simulink model "savareseC2"  (R2023a)
settings: Solver=FixedStepDiscrete  StartTime=0.0  StopTime=200  FixedStep=Ts  MaxStep=Ts  RelTol=1e-3
model workspace (MAT data in the model file):
  Ts = 0.002
  acoeff = 0.95
  amax = 0.1
  jcoeff = 0.1
  jmax = 1
  pf = 160
  reference_command = [0 0.002 0.004 0.006 0.008 0.01 0.012 0.014 0.016 0.018 0.02 0.022 ... (200002 elements, 100001x2)]
  v = 50
  vmax = 1.5
undefined symbols (not defined in the file or in its folder): DiscIntNeverNeededParam
(part 1 of 2)
settings Model: Creator=savar  LastModifiedBy=giaco
settings SolverCC: AlgebraicLoopSolver=TrustRegion
settings DebuggingCC: UnconnectedInputMsg=warning  UnconnectedOutputMsg=warning  UnconnectedLineMsg=warning
settings ModelReferenceCC: EnableRefExpFcnMdlSchedulingChecks=on
settings RTWCC: DLArmComputeVersion=19.05

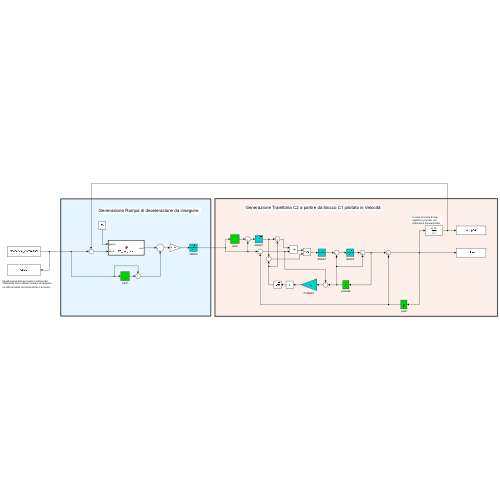
[thumbnail: Simulink's stored preview of the top-level diagram]
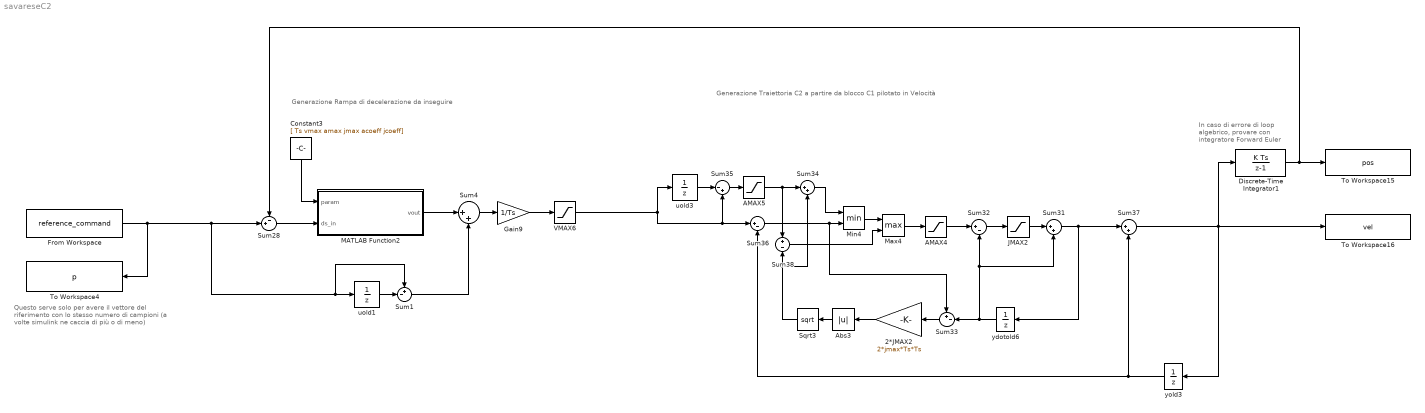
== system savareseC2 ==
  note: Questo serve solo per avere il vettore del riferimento con lo stesso numero di campioni
      | (a volte simulink ne caccia di più o di meno)
  note: In caso di errore di loop algebrico, provare con integratore Forward Euler
  note: Generazione Traiettoria C2 a partire da blocco C1 pilotato in Velocità
  note: Generazione Rampa di decelerazione da inseguire
  2*JMAX2 : Gain  Gain=2*jmax*Ts*Ts
  AMAX4 : Saturate  UpperLimit=amax*Ts  LowerLimit=-amax*Ts
  AMAX5 : Saturate  UpperLimit=amax*Ts  LowerLimit=-amax*Ts
  Abs3 : Abs  SaturateOnIntegerOverflow=off
  Constant3 : Constant  Value=[ Ts vmax amax jmax acoeff jcoeff]
  Discrete-Time Integrator1 : DiscreteIntegrator  SampleTime=-1  ICPrevOutput=DiscIntNeverNeededParam  ICPrevScaledInput=DiscIntNeverNeededParam
  From Workspace : FromWorkspace  VariableName=reference_command
  Gain9 : Gain  Gain=1/Ts
  JMAX2 : Saturate  UpperLimit=jmax*Ts*Ts  LowerLimit=-jmax*Ts*Ts
  MATLAB Function2 : MATLAB Function  TreatAsAtomicUnit=on
  Max4 : MinMax  Function=max  Inputs=2
  Min4 : MinMax  Inputs=2
  Sqrt3 : Sqrt
  Sum1 : Sum  Inputs=+-|
  Sum28 : Sum  Inputs=-+|
  Sum{4,31,34,37} (4 alike) : Sum  Inputs=|++
  Sum32 : Sum  Inputs=|+-
  Sum33 : Sum  Inputs=+-|
  Sum35 : Sum  Inputs=|-+
  Sum36 : Sum  Inputs=|+-
  Sum38 : Sum  Inputs=+-
  To Workspace15 : ToWorkspace  VariableName=pos  SampleTime=-1
      settings: Save2DSignal=2-D array (concatenate along first dimension)
  To Workspace16 : ToWorkspace  VariableName=vel  SampleTime=-1
      settings: Save2DSignal=2-D array (concatenate along first dimension)
  To Workspace4 : ToWorkspace  VariableName=p  SampleTime=-1
      settings: Save2DSignal=2-D array (concatenate along first dimension)
  VMAX6 : Saturate  UpperLimit=vmax  LowerLimit=-vmax
  uold1 : UnitDelay  SampleTime=-1  HasFrameUpgradeWarning=on
  uold3 : UnitDelay  SampleTime=-1  HasFrameUpgradeWarning=on
  ydotold6 : UnitDelay  SampleTime=-1  HasFrameUpgradeWarning=on
  yold3 : UnitDelay  SampleTime=-1  HasFrameUpgradeWarning=on
  wires:
  Constant3/1 -> MATLAB Function2/1(param)
  Sum33/1 -> 2*JMAX2/1
  2*JMAX2/1 -> Abs3/1
  Sum38/1 -> Max4/2
  Abs3/1 -> Sqrt3/1
  Max4/1 -> AMAX4/1
  AMAX5/1 -> Sum34/1, Sum38/1
  uold3/1 -> Sum35/1
  ydotold6/1 -> Sum32/2, Sum31/2, Sum33/2
  yold3/1 -> Sum36/2, Sum37/2
  Min4/1 -> Max4/1
  AMAX4/1 -> Sum32/1
  Sqrt3/1 -> Sum38/2, Sum34/2
  JMAX2/1 -> Sum31/1
  Sum32/1 -> JMAX2/1
  Sum34/1 -> Min4/1
  Sum36/1 -> Sum33/1, Min4/2
  Sum31/1 -> Sum37/1, ydotold6/1
  Sum35/1 -> AMAX5/1
  From Workspace/1 -> To Workspace4/1, Sum28/2, Sum1/1, uold1/1
  Discrete-Time Integrator1/1 -> To Workspace15/1, Sum28/1
  Sum28/1 -> MATLAB Function2/2(ds_in)
  MATLAB Function2/1(vout) -> Sum4/1
  Sum37/1 -> To Workspace16/1, Discrete-Time Integrator1/1, yold3/1
  VMAX6/1 -> Sum35/2, Sum36/1, uold3/1
  Sum4/1 -> Gain9/1
  Gain9/1 -> VMAX6/1
  uold1/1 -> Sum1/2
  Sum1/1 -> Sum4/2
